simulink model "flightControlSystem"  (R2022b)
settings: Solver=ode3  StartTime=0  StopTime=TFinal  FixedStep=Ts  RelTol=1e-3  EnableMultiTasking=on
model workspace (MAT data in the model file):
  D_gain = 0.03
  I_gain = 1.9
  PD_gain = 4e-05
  P_gain = 6
  case0_gain = 0.999
  en = 0.4
  kado_delay = 20
  last_gain = 0.0008
  ririku = 400
  start = 1400
undefined symbols (not defined in the file): codertarget, Controller, DiscIntNeverNeededParam, Discrete, Estimator, g, gray, init, Sensors, Time, Ts, var_acc_angle_N, var_bias_gyr_N, var_gyro_p_N, Vehicle
libraries: simulink x80, visionstatistics x8, sldvlib x7, slpidlib x4, ctrlSharedLib x4, sharedtransform x3, dspstat3 x2, parrotlib x1
(part 2 of 3)

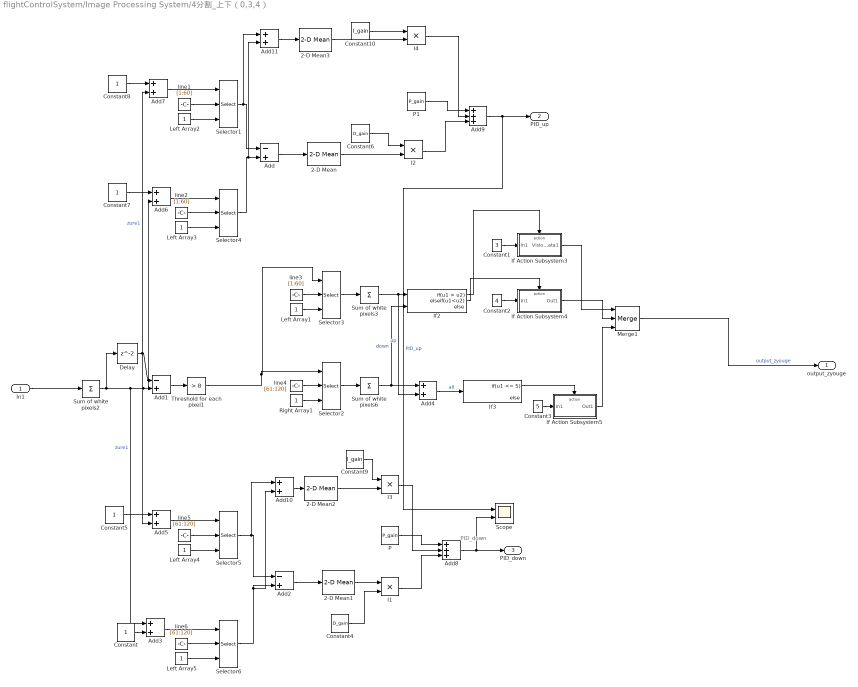
== system flightControlSystem/Image Processing System/4分割_上下（0,3,4） ==
  note: PID_down
  In1 : Inport
  2-D Mean{,1..3} (4 alike) : visionstatistics/2-D Mean  run=off  reset_popup=None  directionMode=Entire input  dimension=1  treatSBRowAsCol=on  outputLastDataTypeStr=Inherit: Same as accumulator  accumMode=Binary point scaling  accumWordLength=32  accumFracLength=0  accumLastDataTypeStr=fixdt([],32,0)  roiEnable=off  roiType=Rectangles  roiPortion=Entire ROI  roiOutput=Individual statistics for each ROI  roiFlag=off  roundingMode=Floor  overflowMode=off  accumDataTypeStr=fixdt([],32,0)  outputDataTypeStr=Inherit: Same as accumulator  outputMin=[]  outputMax=[]
  Add : Sum  Inputs=-+
  Add1 : Sum  Inputs=-+  SaturateOnIntegerOverflow=on
  Add{3..7,10..11} (7 alike) : Sum
  Add2 : Sum  Inputs=-+
  Add8 : Sum  Inputs=+++
  Add9 : Sum  Inputs=+++
  Constant{,5,7..8} (4 alike) : Constant
  Constant1 : Constant  Value=3
  Constant10 : Constant  Value=I_gain
  Constant2 : Constant  Value=4
  Constant3 : Constant  Value=5
  Constant4 : Constant  Value=D_gain
  Constant6 : Constant  Value=D_gain
  Constant9 : Constant  Value=I_gain
  Delay : Delay
  I{1..4} (4 alike) : Product
  If Action Subsystem3 : Subsystem  TreatAsAtomicUnit=on
  If Action Subsystem4 : Subsystem  TreatAsAtomicUnit=on
  If Action Subsystem5 : Subsystem  TreatAsAtomicUnit=on
  If2 : If  NumInputs=2  IfExpression=u1 > u2  ElseIfExpressions=u1<u2
  If3 : If  IfExpression=u1 <= 5
  Left Array{1..5} (5 alike) : Constant  OutMin=[1]
  Merge1 : Merge  Inputs=3  InitialOutput=[0]
  P : Constant  Value=P_gain
  P1 : Constant  Value=P_gain
  Right Array1 : Constant  OutMin=[1]
  Scope : Scope  NumInputPorts=2
  Selector{1..6} (6 alike) : Selector  NumberOfDimensions=2  InputPortWidth=3  IndexOptions=Index vector (port),Index vector (port)  Indices=[1 3],1  OutputSizes=1,1
  Sum of white pixels2 : Sum  Inputs=+  CollapseMode=Specified dimension  CollapseDim=2  OutDataTypeStr=uint16
  Sum of white pixels3 : Sum  Inputs=+  OutDataTypeStr=uint16
  Sum of white pixels6 : Sum  Inputs=+  OutDataTypeStr=uint16
  Threshold for each pixel1 : simulink/Logic and Bit Operations/Compare To Constant  relop=>  const=8  OutDataTypeStr=boolean
  line1 : Constant  Value=[1:60]
  line2 : Constant  Value=[1:60]
  line3 : Constant  Value=[1:60]
  line4 : Constant  Value=[61:120]
  line5 : Constant  Value=[61:120]
  line6 : Constant  Value=[61:120]
  output_zyouge : Outport
  PID_up : Outport  Port=2
  PID_down : Outport  Port=3
  wires:
  Constant3/1 -> If Action Subsystem5/1(In1)
  Merge1/1 -> output_zyouge/1  "output_zyouge"
  Add1/1 -> Threshold for each pixel1/1
  line3/1 -> Selector3/2
  Left Array1/1 -> Selector3/3
  Right Array1/1 -> Selector2/3
  If3/1 -> If Action Subsystem5/Action
  Sum of white pixels3/1 -> If2/1, Add4/1  "up"
  If Action Subsystem5/1(Out1) -> Merge1/3
  Sum of white pixels6/1 -> Add4/2, If2/2  "down"
  Threshold for each pixel1/1 -> Selector2/1, Selector3/1
  line4/1 -> Selector2/2
  If2/1 -> If Action Subsystem3/Action
  Constant2/1 -> If Action Subsystem4/1(In1)
  If2/2 -> If Action Subsystem4/Action
  Selector3/1 -> Sum of white pixels3/1
  If Action Subsystem4/1(Out1) -> Merge1/2
  If Action Subsystem3/1(Vision-based Data1) -> Merge1/1
  Add4/1 -> If3/1  "all"
  Constant1/1 -> If Action Subsystem3/1(In1)
  In1/1 -> Sum of white pixels2/1
  Constant6/1 -> I2/1
  Selector2/1 -> Sum of white pixels6/1
  Constant4/1 -> I1/2
  2-D Mean/1 -> I2/2
  2-D Mean1/1 -> I1/1
  Left Array2/1 -> Selector1/3
  line1/1 -> Selector1/2
  Left Array3/1 -> Selector4/3
  line2/1 -> Selector4/2
  Selector1/1 -> Add11/1, Add/1
  Selector4/1 -> Add11/2, Add/2
  Add/1 -> 2-D Mean/1
  Sum of white pixels2/1 -> Delay/1, Add3/1, Add6/2, Add1/2  "zure1"
  Left Array5/1 -> Selector6/3
  Selector6/1 -> Add10/2, Add2/2
  Selector5/1 -> Add10/1, Add2/1
  Left Array4/1 -> Selector5/3
  Delay/1 -> Add7/2, Add5/2, Add1/1  "zure1"
  line5/1 -> Selector5/2
  line6/1 -> Selector6/2
  Add2/1 -> 2-D Mean1/1
  Add3/1 -> Selector6/1
  Constant/1 -> Add3/2
  Add5/1 -> Selector5/1
  Constant5/1 -> Add5/1
  Add6/1 -> Selector4/1
  Constant7/1 -> Add6/1
  Add7/1 -> Selector1/1
  Constant8/1 -> Add7/1
  Add8/1 -> Scope/2, PID_down/1
  P/1 -> Add8/1
  I1/1 -> Add8/3
  Add9/1 -> Scope/1, PID_up/1  "PID_up"
  P1/1 -> Add9/1
  Add10/1 -> 2-D Mean2/1
  2-D Mean2/1 -> I3/2
  Constant9/1 -> I3/1
  I3/1 -> Add8/2
  Add11/1 -> 2-D Mean3/1
  2-D Mean3/1 -> I4/2
  Constant10/1 -> I4/1
  I4/1 -> Add9/2
  I2/1 -> Add9/3

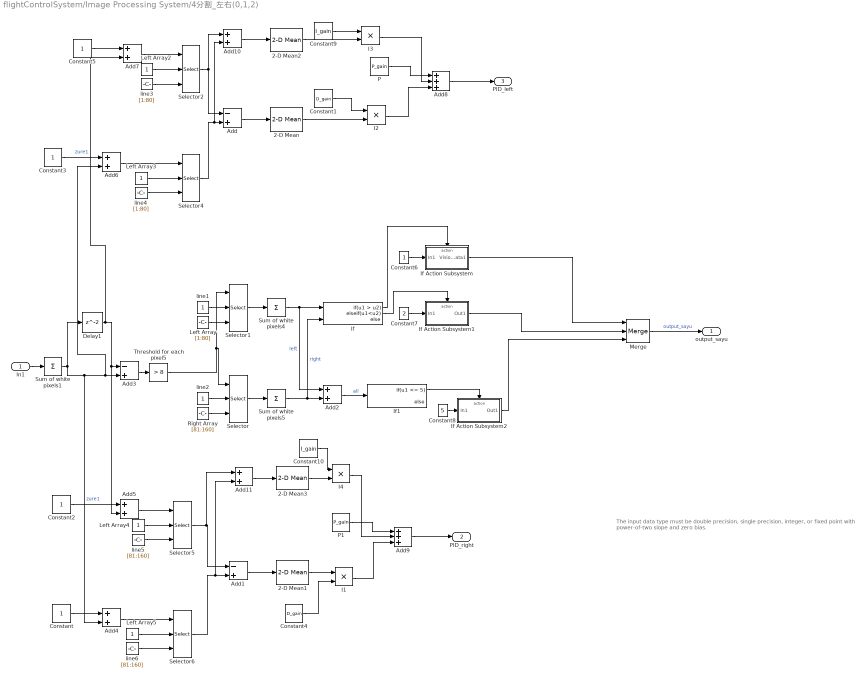
== system flightControlSystem/Image Processing System/4分割_左右(0,1,2) ==
  note: The input data type must be double precision, single precision, integer, or fixed point with power-of-two slope and zero bias.
  In1 : Inport
  2-D Mean{,1..3} (4 alike) : visionstatistics/2-D Mean  run=off  reset_popup=None  directionMode=Entire input  dimension=1  treatSBRowAsCol=on  outputLastDataTypeStr=Inherit: Same as accumulator  accumMode=Binary point scaling  accumWordLength=32  accumFracLength=0  accumLastDataTypeStr=fixdt([],32,0)  roiEnable=off  roiType=Rectangles  roiPortion=Entire ROI  roiOutput=Individual statistics for each ROI  roiFlag=off  roundingMode=Floor  overflowMode=off  accumDataTypeStr=fixdt([],32,0)  outputDataTypeStr=Inherit: Same as accumulator  outputMin=[]  outputMax=[]
  Add : Sum  Inputs=-+
  Add1 : Sum  Inputs=-+
  Add{2,4..7,10..11} (7 alike) : Sum
  Add3 : Sum  Inputs=-+  SaturateOnIntegerOverflow=on
  Add8 : Sum  Inputs=+++
  Add9 : Sum  Inputs=+++
  Constant{,2..3,5..6} (5 alike) : Constant
  Constant1 : Constant  Value=D_gain
  Constant10 : Constant  Value=I_gain
  Constant4 : Constant  Value=D_gain
  Constant7 : Constant  Value=2
  Constant8 : Constant  Value=5
  Constant9 : Constant  Value=I_gain
  Delay1 : Delay
  I{1..4} (4 alike) : Product
  If : If  NumInputs=2  IfExpression=u1 > u2  ElseIfExpressions=u1<u2
  If Action Subsystem : Subsystem  TreatAsAtomicUnit=on
  If Action Subsystem1 : Subsystem  TreatAsAtomicUnit=on
  If Action Subsystem2 : Subsystem  TreatAsAtomicUnit=on
  If1 : If  IfExpression=u1 <= 5
  Left Array : Constant  Value=[1:80]  OutMin=[1]
  Left Array{2..5} (4 alike) : Constant  OutMin=[1]
  Merge : Merge  Inputs=3  InitialOutput=[0]
  P : Constant  Value=P_gain
  P1 : Constant  Value=P_gain
  Right Array : Constant  Value=[81:160]  OutMin=[1]
  Selector{,1..2,4..6} (6 alike) : Selector  NumberOfDimensions=2  InputPortWidth=3  IndexOptions=Index vector (port),Index vector (port)  Indices=[1 3],1  OutputSizes=1,1
  Sum of white pixels1 : Sum  Inputs=+  CollapseMode=Specified dimension  OutDataTypeStr=uint16
  Sum of white pixels4 : Sum  Inputs=+  OutDataTypeStr=uint16
  Sum of white pixels5 : Sum  Inputs=+  OutDataTypeStr=uint16
  Threshold for each pixel5 : simulink/Logic and Bit Operations/Compare To Constant  relop=>  const=8  OutDataTypeStr=boolean
  line1 : Constant
  line2 : Constant
  line3 : Constant  Value=[1:80]
  line4 : Constant  Value=[1:80]
  line5 : Constant  Value=[81:160]
  line6 : Constant  Value=[81:160]
  output_sayu : Outport
  PID_right : Outport  Port=2
  PID_left : Outport  Port=3
  wires:
  If1/1 -> If Action Subsystem2/Action
  Sum of white pixels5/1 -> Add2/2, If/2  "right"
  Constant7/1 -> If Action Subsystem1/1(In1)
  Add3/1 -> Threshold for each pixel5/1
  If Action Subsystem2/1(Out1) -> Merge/3
  line1/1 -> Selector1/2
  If Action Subsystem/1(Vision-based Data1) -> Merge/1
  Right Array/1 -> Selector/3
  Sum of white pixels4/1 -> If/1, Add2/1  "left"
  Threshold for each pixel5/1 -> Selector1/1, Selector/1
  If/1 -> If Action Subsystem/Action
  If/2 -> If Action Subsystem1/Action
  If Action Subsystem1/1(Out1) -> Merge/2
  Constant8/1 -> If Action Subsystem2/1(In1)
  In1/1 -> Sum of white pixels1/1
  Left Array/1 -> Selector1/3
  Constant6/1 -> If Action Subsystem/1(In1)
  line2/1 -> Selector/2
  Add2/1 -> If1/1  "all"
  Merge/1 -> output_sayu/1  "output_sayu"
  Selector1/1 -> Sum of white pixels4/1
  Selector/1 -> Sum of white pixels5/1
  Add/1 -> 2-D Mean/1
  2-D Mean/1 -> I2/2
  Selector4/1 -> Add10/2, Add/2
  Selector2/1 -> Add10/1, Add/1
  Constant1/1 -> I2/1
  Sum of white pixels1/1 -> Add4/2, Add6/2, Add3/2, Delay1/1  "zure1"
  Add1/1 -> 2-D Mean1/1
  Selector6/1 -> Add11/2, Add1/2
  Selector5/1 -> Add11/1, Add1/1
  Delay1/1 -> Add7/2, Add5/2, Add3/1  "zure1"
  2-D Mean1/1 -> I1/1
  Constant4/1 -> I1/2
  Left Array3/1 -> Selector4/2
  line4/1 -> Selector4/3
  Left Array2/1 -> Selector2/2
  line3/1 -> Selector2/3
  Left Array4/1 -> Selector5/2
  line5/1 -> Selector5/3
  Left Array5/1 -> Selector6/2
  line6/1 -> Selector6/3
  Add4/1 -> Selector6/1
  Constant/1 -> Add4/1
  Add5/1 -> Selector5/1
  Constant2/1 -> Add5/1
  Add6/1 -> Selector4/1
  Constant3/1 -> Add6/1
  Add7/1 -> Selector2/1
  Constant5/1 -> Add7/1
  I2/1 -> Add8/3
  Add8/1 -> PID_left/1
  P/1 -> Add8/1
  I1/1 -> Add9/3
  Add9/1 -> PID_right/1
  P1/1 -> Add9/1
  Add10/1 -> 2-D Mean2/1
  2-D Mean2/1 -> I3/2
  Constant9/1 -> I3/1
  I3/1 -> Add8/2
  Add11/1 -> 2-D Mean3/1
  2-D Mean3/1 -> I4/2
  Constant10/1 -> I4/1
  I4/1 -> Add9/2

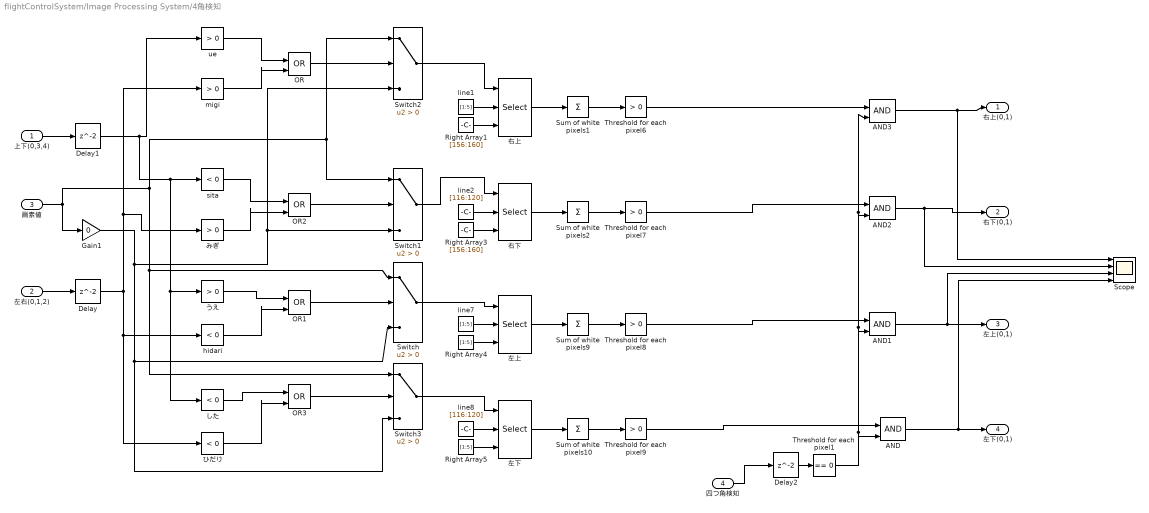
== system flightControlSystem/Image Processing System/4角検知 ==
  上下(0,3,4) : Inport
  左右(0,1,2) : Inport  Port=2
  画素値 : Inport  Port=3
  四つ角検知 : Inport  Port=4
  AND{,1..3} (4 alike) : Logic  IconShape=distinctive  AllPortsSameDT=off  OutDataTypeStr=boolean
  Delay : Delay
  Delay1 : Delay
  Delay2 : Delay
  Gain1 : Gain  Gain=0
  OR{,1..3} (4 alike) : Logic  Operator=OR  IconShape=distinctive  AllPortsSameDT=off  OutDataTypeStr=boolean
  Right Array1 : Constant  Value=[156:160]  OutMin=[1]
  Right Array3 : Constant  Value=[156:160]  OutMin=[1]
  Right Array4 : Constant  Value=[1:5]  OutMin=[1]
  Right Array5 : Constant  Value=[1:5]  OutMin=[1]
  Scope : Scope  NumInputPorts=4
  Sum of white pixels{1..2,9..10} (4 alike) : Sum  Inputs=+  OutDataTypeStr=uint16
  Switch{,1..3} (4 alike) : Switch  Criteria=u2 > Threshold  SaturateOnIntegerOverflow=off  InputSameDT=off
  Threshold for each pixel1 : simulink/Logic and Bit Operations/Compare To Constant  relop===  const=0  OutDataTypeStr=boolean
  Threshold for each pixel{6..9} (4 alike) : simulink/Logic and Bit Operations/Compare To Constant  relop=>  const=0  OutDataTypeStr=boolean
  hidari : simulink/Logic and Bit Operations/Compare To Constant  relop=<  const=0  OutDataTypeStr=boolean
  line1 : Constant  Value=[1:5]
  line2 : Constant  Value=[116:120]
  line7 : Constant  Value=[1:5]
  line8 : Constant  Value=[116:120]
  migi : simulink/Logic and Bit Operations/Compare To Constant  relop=>  const=0  OutDataTypeStr=boolean
  sita : simulink/Logic and Bit Operations/Compare To Constant  relop=<  const=0  OutDataTypeStr=boolean
  ue : simulink/Logic and Bit Operations/Compare To Constant  relop=>  const=0  OutDataTypeStr=boolean
  うえ : simulink/Logic and Bit Operations/Compare To Constant  relop=>  const=0  OutDataTypeStr=boolean
  した : simulink/Logic and Bit Operations/Compare To Constant  relop=<  const=0  OutDataTypeStr=boolean
  ひだり : simulink/Logic and Bit Operations/Compare To Constant  relop=<  const=0  OutDataTypeStr=boolean
  みぎ : simulink/Logic and Bit Operations/Compare To Constant  relop=>  const=0  OutDataTypeStr=boolean
  右上 : Selector  NumberOfDimensions=2  InputPortWidth=3  IndexOptions=Index vector (port),Index vector (port)  Indices=[1 3],1  OutputSizes=1,1
  右下 : Selector  NumberOfDimensions=2  InputPortWidth=3  IndexOptions=Index vector (port),Index vector (port)  Indices=[1 3],1  OutputSizes=1,1
  左上 : Selector  NumberOfDimensions=2  InputPortWidth=3  IndexOptions=Index vector (port),Index vector (port)  Indices=[1 3],1  OutputSizes=1,1
  左下 : Selector  NumberOfDimensions=2  InputPortWidth=3  IndexOptions=Index vector (port),Index vector (port)  Indices=[1 3],1  OutputSizes=1,1
  右上(0,1) : Outport
  右下(0,1) : Outport  Port=2
  左上(0,1) : Outport  Port=3
  左下(0,1) : Outport  Port=4
  wires:
  左下/1 -> Sum of white pixels10/1
  line2/1 -> 右下/2
  Right Array5/1 -> 左下/3
  line8/1 -> 左下/2
  Right Array3/1 -> 右下/3
  line1/1 -> 右上/2
  右上/1 -> Sum of white pixels1/1
  Right Array4/1 -> 左上/3
  右下/1 -> Sum of white pixels2/1
  Sum of white pixels9/1 -> Threshold for each pixel8/1
  左上/1 -> Sum of white pixels9/1
  Sum of white pixels1/1 -> Threshold for each pixel6/1
  Right Array1/1 -> 右上/3
  line7/1 -> 左上/2
  Sum of white pixels2/1 -> Threshold for each pixel7/1
  Threshold for each pixel9/1 -> AND/1
  Sum of white pixels10/1 -> Threshold for each pixel9/1
  Threshold for each pixel7/1 -> AND2/1
  Threshold for each pixel8/1 -> AND1/1
  Threshold for each pixel6/1 -> AND3/1
  AND3/1 -> Scope/1, 右上(0,1)/1
  AND2/1 -> Scope/2, 右下(0,1)/1
  AND1/1 -> Scope/3, 左上(0,1)/1
  AND/1 -> Scope/4, 左下(0,1)/1
  画素値/1 -> Switch3/1, Switch/1, Switch1/1, Switch2/1, Gain1/1
  左右(0,1,2)/1 -> Delay/1
  Switch/1 -> 左上/1
  Switch1/1 -> 右下/1
  ue/1 -> OR/1
  migi/1 -> OR/2
  OR/1 -> Switch2/2
  Switch2/1 -> 右上/1
  上下(0,3,4)/1 -> Delay1/1
  Switch3/1 -> 左下/1
  Delay1/1 -> ue/1, した/1, うえ/1, sita/1
  Delay/1 -> みぎ/1, migi/1, hidari/1, ひだり/1
  Gain1/1 -> Switch1/3, Switch2/3, Switch/3, Switch3/3
  OR2/1 -> Switch1/2
  OR1/1 -> Switch/2
  OR3/1 -> Switch3/2
  ひだり/1 -> OR3/2
  した/1 -> OR3/1
  hidari/1 -> OR1/2
  うえ/1 -> OR1/1
  みぎ/1 -> OR2/2
  sita/1 -> OR2/1
  四つ角検知/1 -> Delay2/1
  Delay2/1 -> Threshold for each pixel1/1
  Threshold for each pixel1/1 -> AND1/2, AND3/2, AND2/2, AND/2

== system flightControlSystem/Image Processing System/If Action Subsystem ==
  In1 : Inport
  Action Port : ActionPort  ActionPortLabel=if(u1 == 0 & u2==5)
  Out1 : Outport
  wires:
  In1/1 -> Out1/1

== system flightControlSystem/Image Processing System/If Action Subsystem1 ==
  In1 : Inport
  Action Port : ActionPort  ActionPortLabel=else
  Out1 : Outport
  wires:
  In1/1 -> Out1/1

== system flightControlSystem/Image Processing System/If Action Subsystem2 ==
  In1 : Inport  OutDataTypeStr=double
  Action Port : ActionPort  ActionPortLabel=if(u1 == 0 & u2==5)
  Out1 : Outport
  wires:
  In1/1 -> Out1/1

== system flightControlSystem/Image Processing System/If Action Subsystem3 ==
  In1 : Inport
  Action Port : ActionPort  ActionPortLabel=else
  Out1 : Outport
  wires:
  In1/1 -> Out1/1

== system flightControlSystem/Image Processing System/Switch Case Action Subsystem ==
  In1 : Inport
  Action Port : ActionPort  ActionPortLabel=case [ 0 ]:
  Out1 : Outport
  wires:
  In1/1 -> Out1/1

== system flightControlSystem/Image Processing System/Switch Case Action Subsystem1 ==
  In1 : Inport
  Action Port : ActionPort  ActionPortLabel=case [ 7 ]:
  Out1 : Outport
  wires:
  In1/1 -> Out1/1

== system flightControlSystem/Image Processing System/Switch Case Action Subsystem2 ==
  In1 : Inport
  Action Port : ActionPort  ActionPortLabel=case [ 3 ]:
  Out1 : Outport
  wires:
  In1/1 -> Out1/1

== system flightControlSystem/Image Processing System/Switch Case Action Subsystem3 ==
  In1 : Inport
  Action Port : ActionPort  ActionPortLabel=case [ 4 ]:
  Out1 : Outport
  wires:
  In1/1 -> Out1/1

== system flightControlSystem/Image Processing System/Switch Case Action Subsystem4 ==
  In1 : Inport
  Action Port : ActionPort  ActionPortLabel=case [ 3 ]:
  Out1 : Outport
  wires:
  In1/1 -> Out1/1

== system flightControlSystem/Image Processing System/Switch Case Action Subsystem5 ==
  In1 : Inport
  Action Port : ActionPort  ActionPortLabel=case [ 2 ]:
  Out1 : Outport
  wires:
  In1/1 -> Out1/1

== system flightControlSystem/Image Processing System/Switch Case Action Subsystem6 ==
  In1 : Inport
  Action Port : ActionPort  ActionPortLabel=case [ 1 ]:
  Out1 : Outport
  wires:
  In1/1 -> Out1/1

== system flightControlSystem/Image Processing System/Switch Case Action Subsystem7 ==
  In1 : Inport
  Action Port : ActionPort  ActionPortLabel=case [ 0 ]:
  Out1 : Outport
  wires:
  In1/1 -> Out1/1

== system flightControlSystem/Image Processing System/外枠検知 ==
  In1 : Inport
  Right Array1 : Constant  Value=[1:160]  OutMin=[1]
  Right Array3 : Constant  Value=[1:160]  OutMin=[1]
  Right Array4 : Constant  Value=[120:160]  OutMin=[1]
  Right Array5 : Constant  Value=[1:40]  OutMin=[1]
  Sum of white pixels{1..2,9..10} (4 alike) : Sum  Inputs=+  OutDataTypeStr=uint16
  Threshold for each pixel{6..9} (4 alike) : simulink/Logic and Bit Operations/Compare To Constant  relop=<=  const=5  OutDataTypeStr=boolean
  line1 : Constant  Value=[1:30]
  line2 : Constant  Value=[90:120]
  line7 : Constant  Value=[1:120]
  line8 : Constant  Value=[1:120]
  上上 : Selector  NumberOfDimensions=2  InputPortWidth=3  IndexOptions=Index vector (port),Index vector (port)  Indices=[1 3],1  OutputSizes=1,1
  下下 : Selector  NumberOfDimensions=2  InputPortWidth=3  IndexOptions=Index vector (port),Index vector (port)  Indices=[1 3],1  OutputSizes=1,1
  右右 : Selector  NumberOfDimensions=2  InputPortWidth=3  IndexOptions=Index vector (port),Index vector (port)  Indices=[1 3],1  OutputSizes=1,1
  左左 : Selector  NumberOfDimensions=2  InputPortWidth=3  IndexOptions=Index vector (port),Index vector (port)  Indices=[1 3],1  OutputSizes=1,1
  y : Outport
  y1 : Outport  Port=2
  y2 : Outport  Port=3
  y3 : Outport  Port=4
  wires:
  line1/1 -> 上上/2
  上上/1 -> Sum of white pixels1/1
  Sum of white pixels1/1 -> Threshold for each pixel6/1
  In1/1 -> 右右/1, 左左/1, 下下/1, 上上/1
  Sum of white pixels2/1 -> Threshold for each pixel7/1
  Sum of white pixels9/1 -> Threshold for each pixel8/1
  左左/1 -> Sum of white pixels10/1
  Threshold for each pixel6/1 -> y/1
  line8/1 -> 左左/2
  line7/1 -> 右右/2
  Sum of white pixels10/1 -> Threshold for each pixel9/1
  右右/1 -> Sum of white pixels9/1
  Right Array1/1 -> 上上/3
  Right Array4/1 -> 右右/3
  line2/1 -> 下下/2
  Threshold for each pixel7/1 -> y1/1
  下下/1 -> Sum of white pixels2/1
  Threshold for each pixel9/1 -> y2/1
  Right Array3/1 -> 下下/3
  Right Array5/1 -> 左左/3
  Threshold for each pixel8/1 -> y3/1

== system flightControlSystem/Image Processing System/論理回路 ==
  In1 : Inport
  In2 : Inport  Port=2
  In3 : Inport  Port=3
  In4 : Inport  Port=4
  AND{,1..3} (4 alike) : Logic  Inputs=4  IconShape=distinctive  AllPortsSameDT=off  OutDataTypeStr=boolean
  NOT{,1..3} (4 alike) : Logic  Operator=NOT  IconShape=distinctive  AllPortsSameDT=off  OutDataTypeStr=boolean
  OR : Logic  Operator=OR  Inputs=4  IconShape=distinctive  AllPortsSameDT=off  OutDataTypeStr=boolean
  Out1 : Outport
  wires:
  In1/1 -> AND/1, NOT/1
  In2/1 -> AND1/2, NOT1/1
  In3/1 -> AND2/3, NOT2/1
  In4/1 -> AND3/4, NOT3/1
  NOT/1 -> AND2/1, AND1/1, AND3/1
  NOT1/1 -> AND3/2, AND2/2, AND/2
  NOT2/1 -> AND3/3, AND/3, AND1/3
  NOT3/1 -> AND2/4, AND1/4, AND/4
  AND/1 -> OR/1
  AND1/1 -> OR/2
  AND2/1 -> OR/3
  AND3/1 -> OR/4
  OR/1 -> Out1/1

== system flightControlSystem/Control System/Controller/Altitude Controller ==
  note: PID Controller for Altitude
  note: ALTITUDE CONTROLLER
  states_estim : Inport
  PosZ : Inport  Port=2
  takeoff_flag : Inport  Port=3
  Bus Selector1 : BusSelector  OutputSignals=Z,dz
  Compare To Constant : simulink/Logic and Bit Operations/Compare To Constant  relop=<  const=100  OutDataTypeStr=boolean
  Counter Free-Running : simulink/Sources/Counter Free-Running  NumBits=16  tsamp=-1
  D_z1 : Gain  Gain=0.5  ParamDataTypeStr=single  OutDataTypeStr=single  SaturateOnIntegerOverflow=on
  Discrete-Time Integrator : DiscreteIntegrator  ExternalReset=falling  SampleTime=Ts  LimitOutput=on  UpperSaturationLimit=2  LowerSaturationLimit=-2  ICPrevOutput=DiscIntNeverNeededParam  ICPrevScaledInput=DiscIntNeverNeededParam
  I_pr : Gain  Gain=0.24
  P_z1 : Gain  Gain=0.8  ParamDataTypeStr=single  OutDataTypeStr=single  SaturateOnIntegerOverflow=on
  SaturationThrust1 : Saturate  UpperLimit=4*Controller.totalThrustMaxRelative*Controller.motorsThrustPerMotorMax  LowerLimit=-4*Controller.totalThrustMaxRelative*Controller.motorsThrustPerMotorMax  OutDataTypeStr=single
  Sum1 : Sum  Inputs=++-  AccumDataTypeStr=single  OutDataTypeStr=single  SaturateOnIntegerOverflow=on
  Sum2 : Sum  Inputs=+-|  AccumDataTypeStr=single  OutDataTypeStr=single  SaturateOnIntegerOverflow=on
  Sum5 : Sum  Inputs=++|  AccumDataTypeStr=single  OutDataTypeStr=single  SaturateOnIntegerOverflow=on
  TakeoffOrControl_Switch1 : Switch  Criteria=u2 > Threshold  SaturateOnIntegerOverflow=off  InputSameDT=off
  Terminator : Terminator
  takeoff_gain1 : Gain  Gain=Controller.takeoffGain  ParamDataTypeStr=single  OutDataTypeStr=single  SaturateOnIntegerOverflow=on
  w1 : Constant  Value=-g*Vehicle.Airframe.mass  OutDataTypeStr=single  SampleTime=Ts
  altitude_cmd : Outport  VectorParamsAs1DForOutWhenUnconnected=off
  wires:
  TakeoffOrControl_Switch1/1 -> Sum5/2
  Discrete-Time Integrator/1 -> Sum1/1
  PosZ/1 -> Sum2/1
  takeoff_flag/1 -> Terminator/1
  w1/1 -> Sum5/1, takeoff_gain1/1  "Feed forward term to  compensate for gravity"
  P_z1/1 -> Sum1/2
  Counter Free-Running/1 -> Compare To Constant/1
  Bus Selector1/2 -> D_z1/1  "<dz>"
  Sum5/1 -> SaturationThrust1/1
  Bus Selector1/1 -> Sum2/2  "<Z>"
  D_z1/1 -> Sum1/3  "dz"
  Sum1/1 -> TakeoffOrControl_Switch1/3
  Compare To Constant/1 -> Discrete-Time Integrator/2, TakeoffOrControl_Switch1/2
  takeoff_gain1/1 -> TakeoffOrControl_Switch1/1
  states_estim/1 -> Bus Selector1/1
  Sum2/1 -> I_pr/1, P_z1/1  "pitch/roll error"
  I_pr/1 -> Discrete-Time Integrator/1
  SaturationThrust1/1 -> altitude_cmd/1

== system flightControlSystem/Control System/Controller/Attitude Controller ==
  note: Inner loop PID
      | controls angular velocity
  note: Outer Proportional loop
      | controls the pitch and roll angle
  note: ATTITUDE CONTROL
  refAttitude : Inport
  states_estim : Inport  Port=2
  Angle control loop : slpidlib/PID Controller  Controller=P  Form=Parallel  TimeDomain=Discrete-time  UseExternalTs=off  SampleTime=Ts  IntegratorMethod=Forward Euler  FilterMethod=Forward Euler  ControllerParametersSource=internal  P=4  I=1  UseKiTs=off  D=0  N=100  UseFilter=on  TunerSelectOption=Transfer Function Based (PID Tuner App)  InitialConditionSource=internal  InitialConditionForIntegrator=0  InitialConditionForFilter=0  DifferentiatorICPrevScaledInput=0  ExternalReset=none  TrackingMode=off  Kt=1  LimitOutput=off  SatLimitsSource=internal  UpperSaturationLimit=inf  LowerSaturationLimit=-inf  LinearizeAsGain=on  AntiWindupMode=none  Kb=1  LimitIntegrator=off  UpperIntegratorSaturationLimit=inf  LowerIntegratorSaturationLimit=-inf  POutMin=[]  POutMax=[]  IOutMin=[]  IOutMax=[]  DOutMin=[]  DOutMax=[]  NOutMin=[]  NOutMax=[]  SumOutMin=[]  SumOutMax=[]  SaturationOutMin=[]  SaturationOutMax=[]  PParamMin=[]  PParamMax=[]  IParamMin=[]  IParamMax=[]  DParamMin=[]  DParamMax=[]  NParamMin=[]  NParamMax=[]  KbParamMin=[]  KbParamMax=[]  KtParamMin=[]  KtParamMax=[]  KbOutMin=[]  KbOutMax=[]  KtOutMin=[]  KtOutMax=[]  IntegratorOutMin=[]  IntegratorOutMax=[]  FilterOutMin=[]  FilterOutMax=[]  SumI1OutMin=[]  SumI1OutMax=[]  SumI2OutMin=[]  SumI2OutMax=[]  SumI3OutMin=[]  SumI3OutMax=[]  SumI4OutMin=[]  SumI4OutMax=[]  SumDOutMin=[]  SumDOutMax=[]  DifferentiatorOutMin=[]  DifferentiatorOutMax=[]  FilterDiffOutCoefMin=[]  FilterDiffOutCoefMax=[]  ReciprocalOutMin=[]  ReciprocalOutMax=[]  SumDenOutMin=[]  SumDenOutMax=[]  SumNumOutMin=[]  SumNumOutMax=[]  DivideOutMin=[]  DivideOutMax=[]  UdiffTsProdOutMin=[]  UdiffTsProdOutMax=[]  NTsProdOutMin=[]  NTsProdOutMax=[]  UintegralTsProdOutMin=[]  UintegralTsProdOutMax=[]  UngainTsProdOutMin=[]  UngainTsProdOutMax=[]  ClampingZeroOutDataTypeStr=Inherit: Inherit via back propagation  ClampingZeroOutMin=[]  ClampingZeroOutMax=[]  FilterDenConstantOutDataTypeStr=Inherit: Inherit via back propagation  FilterDenConstantOutMin=[]  FilterDenConstantOutMax=[]  PCopyOutDataTypeStr=Inherit: Inherit via back propagation  PCopyOutMin=[]  PCopyOutMax=[]  NCopyOutDataTypeStr=Inherit: Inherit via back propagation  NCopyOutMin=[]  NCopyOutMax=[]  IntegratorContinuousStateAttributes=''  IntegratorStateMustResolveToSignalObject=off  IntegratorRTWStateStorageClass=Auto  FilterContinuousStateAttributes=''  FilterStateMustResolveToSignalObject=off  FilterRTWStateStorageClass=Auto  ParallelPVariant=InternalParameters  IdealPVariant=Disabled  IVariant=Disabled  DVariant=Disabled  IntegratorVariant=Disabled  SatVariant=Disabled  AWVariant=Disabled  PCopyVariant=Disabled  TRVariant=Disabled  FdbkBlocksVariant=Forward  IdealPFdbkVariant=Disabled  SatFdbkVariant=Disabled  DerivativeFilterVariant=Disabled  NVariant=Disabled  NCopyVariant=Disabled_SignalSpec  FilterICVariant=Disabled  IntegratorICVariant=Disabled  ExternalResetVariant=Disabled  TRSumVariant=Passthrough  SumFdbkVariant=Disabled  SumVariant=Passthrough_P  TsampFilterVariant=InternalTs  TsampNgainVariant=Passthrough  TsampIntegralVariant=Disabled_SignalSpec  ExternalSaturationOutDataTypeStr=Inherit: Same as second input
  Angular velocity control loop : slpidlib/PID Controller  Controller=PID  Form=Parallel  TimeDomain=Discrete-time  UseExternalTs=off  SampleTime=Ts  IntegratorMethod=Forward Euler  FilterMethod=Forward Euler  ControllerParametersSource=internal  P=0.003*[1 0.81]  I=2*0.003*[1 0.81]  UseKiTs=off  D=0.003/25*[1 0.81]  N=70*[1 1]  UseFilter=on  TunerSelectOption=Transfer Function Based (PID Tuner App)  InitialConditionSource=internal  InitialConditionForIntegrator=0  InitialConditionForFilter=0  DifferentiatorICPrevScaledInput=0  ExternalReset=none  TrackingMode=off  Kt=1  LimitOutput=on  SatLimitsSource=internal  UpperSaturationLimit=0.02  LowerSaturationLimit=-0.02  LinearizeAsGain=on  AntiWindupMode=clamping  Kb=1  LimitIntegrator=off  UpperIntegratorSaturationLimit=inf  LowerIntegratorSaturationLimit=-inf  POutMin=[]  POutMax=[]  IOutMin=[]  IOutMax=[]  DOutMin=[]  DOutMax=[]  NOutMin=[]  NOutMax=[]  SumOutMin=[]  SumOutMax=[]  SaturationOutMin=[]  SaturationOutMax=[]  PParamMin=[]  PParamMax=[]  IParamMin=[]  IParamMax=[]  DParamMin=[]  DParamMax=[]  NParamMin=[]  NParamMax=[]  KbParamMin=[]  KbParamMax=[]  KtParamMin=[]  KtParamMax=[]  KbOutMin=[]  KbOutMax=[]  KtOutMin=[]  KtOutMax=[]  IntegratorOutMin=[]  IntegratorOutMax=[]  FilterOutMin=[]  FilterOutMax=[]  SumI1OutMin=[]  SumI1OutMax=[]  SumI2OutMin=[]  SumI2OutMax=[]  SumI3OutMin=[]  SumI3OutMax=[]  SumI4OutMin=[]  SumI4OutMax=[]  SumDOutMin=[]  SumDOutMax=[]  DifferentiatorOutMin=[]  DifferentiatorOutMax=[]  FilterDiffOutCoefMin=[]  FilterDiffOutCoefMax=[]  ReciprocalOutMin=[]  ReciprocalOutMax=[]  SumDenOutMin=[]  SumDenOutMax=[]  SumNumOutMin=[]  SumNumOutMax=[]  DivideOutMin=[]  DivideOutMax=[]  UdiffTsProdOutMin=[]  UdiffTsProdOutMax=[]  NTsProdOutMin=[]  NTsProdOutMax=[]  UintegralTsProdOutMin=[]  UintegralTsProdOutMax=[]  UngainTsProdOutMin=[]  UngainTsProdOutMax=[]  ClampingZeroOutDataTypeStr=Inherit: Inherit via back propagation  ClampingZeroOutMin=[]  ClampingZeroOutMax=[]  FilterDenConstantOutDataTypeStr=Inherit: Inherit via back propagation  FilterDenConstantOutMin=[]  FilterDenConstantOutMax=[]  PCopyOutDataTypeStr=Inherit: Inherit via back propagation  PCopyOutMin=[]  PCopyOutMax=[]  NCopyOutDataTypeStr=Inherit: Inherit via back propagation  NCopyOutMin=[]  NCopyOutMax=[]  IntegratorContinuousStateAttributes=''  IntegratorStateMustResolveToSignalObject=off  IntegratorRTWStateStorageClass=Auto  FilterContinuousStateAttributes=''  FilterStateMustResolveToSignalObject=off  FilterRTWStateStorageClass=Auto  ParallelPVariant=InternalParameters  IdealPVariant=Disabled  IVariant=InternalParameters  DVariant=InternalParameters  IntegratorVariant=Discrete  SatVariant=Enabled  AWVariant=DiscClampingParallel  PCopyVariant=Disabled  TRVariant=Disabled  FdbkBlocksVariant=Forward  IdealPFdbkVariant=Disabled  SatFdbkVariant=Disabled  DerivativeFilterVariant=ForwardEulerFilter  NVariant=InternalParameters  NCopyVariant=Disabled  FilterICVariant=InternalICsFilter  IntegratorICVariant=InternalICs  ExternalResetVariant=Disabled  TRSumVariant=Passthrough  SumFdbkVariant=Disabled  SumVariant=Sum_PID  TsampFilterVariant=InternalTs  TsampNgainVariant=Passthrough  TsampIntegralVariant=Passthrough  ExternalSaturationOutDataTypeStr=Inherit: Same as second input
  Bus Selector1 : BusSelector  OutputSignals=q,p
  Bus Selector3 : BusSelector  OutputSignals=pitch,roll
  Demux1 : Demux  Outputs=2
  Mux : Mux  Inputs=2
  Mux2 : Mux  Inputs=2
  Sum1 : Sum  Inputs=|+-
  Sum19 : Sum  Inputs=|+-
  tau_pitch : Outport  VectorParamsAs1DForOutWhenUnconnected=off
  tau_roll : Outport  Port=2  VectorParamsAs1DForOutWhenUnconnected=off
  wires:
  Sum1/1 -> Angular velocity control loop/1  "pitch/roll error"
  Angle control loop/1 -> Sum1/1
  Mux2/1 -> Sum1/2
  Sum19/1 -> Angle control loop/1  "pitch/roll error"
  Angular velocity control loop/1 -> Demux1/1
  Demux1/2 -> tau_roll/1  "tau_roll"
  Demux1/1 -> tau_pitch/1  "tau_pitch"
  Bus Selector3/2 -> Mux/2  "<roll>"
  Mux/1 -> Sum19/2
  refAttitude/1 -> Sum19/1
  states_estim/1 -> Bus Selector1/1, Bus Selector3/1
  Bus Selector3/1 -> Mux/1  "<pitch>"
  Bus Selector1/1 -> Mux2/1  "<q>"
  Bus Selector1/2 -> Mux2/2  "<p>"

== system flightControlSystem/Control System/Controller/ControlMixer ==
  tau_pitch : Inport
  tau_roll : Inport  Port=2
  tau_yaw : Inport  Port=3
  totalThrust : Inport  Port=4
  Add : Sum
  Manual Switch : ManualSwitch
  Mux2 : Mux
  Pitch correction : Constant  Value=0.002  OutDataTypeStr=single
  Product : Product  Multiplication=Matrix(*)  RndMeth=Zero
  TorqueTotalThrustToThrustPerMotor : Constant  Value=Controller.Q2Ts  OutDataTypeStr=single
  Variant Source : VariantSource  VariantControlMode=sim codegen switching  VariantActivationTime=update diagram analyze all choices  ShowConditionOnBlock=on
  zero correction : Constant  Value=0  OutDataTypeStr=single
  thrusts_refout : Outport  VectorParamsAs1DForOutWhenUnconnected=off
  wires:
  Product/1 -> thrusts_refout/1
  tau_roll/1 -> Mux2/4
  Add/1 -> Variant Source/2
  tau_yaw/1 -> Mux2/2
  totalThrust/1 -> Mux2/1
  TorqueTotalThrustToThrustPerMotor/1 -> Product/1
  Mux2/1 -> Product/2
  Variant Source/1 -> Mux2/3
  tau_pitch/1 -> Add/1, Variant Source/1
  Pitch correction/1 -> Manual Switch/1
  zero correction/1 -> Manual Switch/2
  Manual Switch/1 -> Add/2

== system flightControlSystem/Control System/Controller/Position Controller ==
  note: Position controller requires good estimate of Yaw orientation to work properly.
      | Incase position control is not needed, the outer loop can be removed and velocity setpoint can be given directly
  note: Inner loop controls linear velocity error
  note: Outer loop controls the position error
  posXY : Inport
  states_estim : Inport  Port=2
  Bus Selector1 : BusSelector  OutputSignals=X,Y
  Bus Selector2 : BusSelector  OutputSignals=dx,dy
  Bus Selector3 : BusSelector  OutputSignals=yaw
  Gain : Gain  Gain=[-1, 1]
  LPF 8Hz Cutoff Filter to avoid oscillations induced by position controller : DiscreteTransferFcn  Numerator=[1, 1]  Denominator=[1+1/pi/Ts/8, 1-1/pi/Ts/8]
  Mux : Mux  Inputs=2
  Mux1 : Mux  Inputs=2
  Position controller : slpidlib/PID Controller  Controller=P  Form=Parallel  TimeDomain=Discrete-time  UseExternalTs=off  SampleTime=Ts  IntegratorMethod=Forward Euler  FilterMethod=Forward Euler  ControllerParametersSource=internal  P=0.7  I=0.1  UseKiTs=off  D=0  N=100  UseFilter=on  TunerSelectOption=Transfer Function Based (PID Tuner App)  InitialConditionSource=internal  InitialConditionForIntegrator=0  InitialConditionForFilter=0  DifferentiatorICPrevScaledInput=0  ExternalReset=none  TrackingMode=off  Kt=1  LimitOutput=on  SatLimitsSource=internal  UpperSaturationLimit=0.5  LowerSaturationLimit=-0.5  LinearizeAsGain=on  AntiWindupMode=clamping  Kb=1  LimitIntegrator=off  UpperIntegratorSaturationLimit=inf  LowerIntegratorSaturationLimit=-inf  POutMin=[]  POutMax=[]  IOutMin=[]  IOutMax=[]  DOutMin=[]  DOutMax=[]  NOutMin=[]  NOutMax=[]  SumOutMin=[]  SumOutMax=[]  SaturationOutMin=[]  SaturationOutMax=[]  PParamMin=[]  PParamMax=[]  IParamMin=[]  IParamMax=[]  DParamMin=[]  DParamMax=[]  NParamMin=[]  NParamMax=[]  KbParamMin=[]  KbParamMax=[]  KtParamMin=[]  KtParamMax=[]  KbOutMin=[]  KbOutMax=[]  KtOutMin=[]  KtOutMax=[]  IntegratorOutMin=[]  IntegratorOutMax=[]  FilterOutMin=[]  FilterOutMax=[]  SumI1OutMin=[]  SumI1OutMax=[]  SumI2OutMin=[]  SumI2OutMax=[]  SumI3OutMin=[]  SumI3OutMax=[]  SumI4OutMin=[]  SumI4OutMax=[]  SumDOutMin=[]  SumDOutMax=[]  DifferentiatorOutMin=[]  DifferentiatorOutMax=[]  FilterDiffOutCoefMin=[]  FilterDiffOutCoefMax=[]  ReciprocalOutMin=[]  ReciprocalOutMax=[]  SumDenOutMin=[]  SumDenOutMax=[]  SumNumOutMin=[]  SumNumOutMax=[]  DivideOutMin=[]  DivideOutMax=[]  UdiffTsProdOutMin=[]  UdiffTsProdOutMax=[]  NTsProdOutMin=[]  NTsProdOutMax=[]  UintegralTsProdOutMin=[]  UintegralTsProdOutMax=[]  UngainTsProdOutMin=[]  UngainTsProdOutMax=[]  ClampingZeroOutDataTypeStr=Inherit: Inherit via back propagation  ClampingZeroOutMin=[]  ClampingZeroOutMax=[]  FilterDenConstantOutDataTypeStr=Inherit: Inherit via back propagation  FilterDenConstantOutMin=[]  FilterDenConstantOutMax=[]  PCopyOutDataTypeStr=Inherit: Inherit via back propagation  PCopyOutMin=[]  PCopyOutMax=[]  NCopyOutDataTypeStr=Inherit: Inherit via back propagation  NCopyOutMin=[]  NCopyOutMax=[]  IntegratorContinuousStateAttributes=''  IntegratorStateMustResolveToSignalObject=off  IntegratorRTWStateStorageClass=Auto  FilterContinuousStateAttributes=''  FilterStateMustResolveToSignalObject=off  FilterRTWStateStorageClass=Auto  ParallelPVariant=InternalParameters  IdealPVariant=Disabled  IVariant=Disabled  DVariant=Disabled  IntegratorVariant=Disabled  SatVariant=Enabled  AWVariant=Disabled  PCopyVariant=Disabled  TRVariant=Disabled  FdbkBlocksVariant=Forward  IdealPFdbkVariant=Disabled  SatFdbkVariant=Disabled  DerivativeFilterVariant=Disabled  NVariant=Disabled  NCopyVariant=Disabled_SignalSpec  FilterICVariant=Disabled  IntegratorICVariant=Disabled  ExternalResetVariant=Disabled  TRSumVariant=Passthrough  SumFdbkVariant=Disabled  SumVariant=Passthrough_P  TsampFilterVariant=InternalTs  TsampNgainVariant=Passthrough  TsampIntegralVariant=Disabled_SignalSpec  ExternalSaturationOutDataTypeStr=Inherit: Same as second input
  Position error transformation (Earth to Body frame) : MATLAB Function  TreatAsAtomicUnit=on
  Sum1 : Sum  Inputs=|+-
  Sum19 : Sum  Inputs=|+-
  Velocity controller : slpidlib/PID Controller  Controller=PI  Form=Parallel  TimeDomain=Discrete-time  UseExternalTs=off  SampleTime=Ts  IntegratorMethod=Forward Euler  FilterMethod=Forward Euler  ControllerParametersSource=internal  P=0.2  I=0.1  UseKiTs=off  D=0  N=100  UseFilter=on  TunerSelectOption=Transfer Function Based (PID Tuner App)  InitialConditionSource=internal  InitialConditionForIntegrator=0  InitialConditionForFilter=0  DifferentiatorICPrevScaledInput=0  ExternalReset=none  TrackingMode=off  Kt=1  LimitOutput=on  SatLimitsSource=internal  UpperSaturationLimit=20*pi/180  LowerSaturationLimit=-20*pi/180  LinearizeAsGain=on  AntiWindupMode=clamping  Kb=1  LimitIntegrator=off  UpperIntegratorSaturationLimit=inf  LowerIntegratorSaturationLimit=-inf  POutMin=[]  POutMax=[]  IOutMin=[]  IOutMax=[]  DOutMin=[]  DOutMax=[]  NOutMin=[]  NOutMax=[]  SumOutMin=[]  SumOutMax=[]  SaturationOutMin=[]  SaturationOutMax=[]  PParamMin=[]  PParamMax=[]  IParamMin=[]  IParamMax=[]  DParamMin=[]  DParamMax=[]  NParamMin=[]  NParamMax=[]  KbParamMin=[]  KbParamMax=[]  KtParamMin=[]  KtParamMax=[]  KbOutMin=[]  KbOutMax=[]  KtOutMin=[]  KtOutMax=[]  IntegratorOutMin=[]  IntegratorOutMax=[]  FilterOutMin=[]  FilterOutMax=[]  SumI1OutMin=[]  SumI1OutMax=[]  SumI2OutMin=[]  SumI2OutMax=[]  SumI3OutMin=[]  SumI3OutMax=[]  SumI4OutMin=[]  SumI4OutMax=[]  SumDOutMin=[]  SumDOutMax=[]  DifferentiatorOutMin=[]  DifferentiatorOutMax=[]  FilterDiffOutCoefMin=[]  FilterDiffOutCoefMax=[]  ReciprocalOutMin=[]  ReciprocalOutMax=[]  SumDenOutMin=[]  SumDenOutMax=[]  SumNumOutMin=[]  SumNumOutMax=[]  DivideOutMin=[]  DivideOutMax=[]  UdiffTsProdOutMin=[]  UdiffTsProdOutMax=[]  NTsProdOutMin=[]  NTsProdOutMax=[]  UintegralTsProdOutMin=[]  UintegralTsProdOutMax=[]  UngainTsProdOutMin=[]  UngainTsProdOutMax=[]  ClampingZeroOutDataTypeStr=Inherit: Inherit via back propagation  ClampingZeroOutMin=[]  ClampingZeroOutMax=[]  FilterDenConstantOutDataTypeStr=Inherit: Inherit via back propagation  FilterDenConstantOutMin=[]  FilterDenConstantOutMax=[]  PCopyOutDataTypeStr=Inherit: Inherit via back propagation  PCopyOutMin=[]  PCopyOutMax=[]  NCopyOutDataTypeStr=Inherit: Inherit via back propagation  NCopyOutMin=[]  NCopyOutMax=[]  IntegratorContinuousStateAttributes=''  IntegratorStateMustResolveToSignalObject=off  IntegratorRTWStateStorageClass=Auto  FilterContinuousStateAttributes=''  FilterStateMustResolveToSignalObject=off  FilterRTWStateStorageClass=Auto  ParallelPVariant=InternalParameters  IdealPVariant=Disabled  IVariant=InternalParameters  DVariant=Disabled  IntegratorVariant=Discrete  SatVariant=Enabled  AWVariant=DiscClampingParallel  PCopyVariant=Disabled  TRVariant=Disabled  FdbkBlocksVariant=Forward  IdealPFdbkVariant=Disabled  SatFdbkVariant=Disabled  DerivativeFilterVariant=Disabled  NVariant=Disabled  NCopyVariant=Disabled_SignalSpec  FilterICVariant=Disabled  IntegratorICVariant=InternalICs  ExternalResetVariant=Disabled  TRSumVariant=Passthrough  SumFdbkVariant=Disabled  SumVariant=Sum_PI  TsampFilterVariant=InternalTs  TsampNgainVariant=Passthrough  TsampIntegralVariant=Passthrough  ExternalSaturationOutDataTypeStr=Inherit: Same as second input
  pitch_roll_cmd : Outport  VectorParamsAs1DForOutWhenUnconnected=off
  wires:
  Bus Selector2/1 -> Mux1/1  "<dx>"
  states_estim/1 -> Bus Selector2/1, Bus Selector3/1, Bus Selector1/1
  Bus Selector1/1 -> Mux/1  "<X>"
  Bus Selector1/2 -> Mux/2  "<Y>"
  Bus Selector2/2 -> Mux1/2  "<dy>"
  Mux1/1 -> Sum19/2
  Sum19/1 -> Velocity controller/1
  Velocity controller/1 -> LPF 8Hz Cutoff Filter to avoid oscillations induced by position controller/1
  Gain/1 -> pitch_roll_cmd/1  "Pitch,Roll setpoint"
  LPF 8Hz Cutoff Filter to avoid oscillations induced by position controller/1 -> Gain/1
  Position controller/1 -> Sum19/1  "Velocity  setpoint"
  Mux/1 -> Sum1/2
  Sum1/1 -> Position error transformation (Earth to Body frame)/2(xy_err_earth)
  Position error transformation (Earth to Body frame)/1(xy_err_body) -> Position controller/1
  posXY/1 -> Sum1/1  "Position setpoint"
  Bus Selector3/1 -> Position error transformation (Earth to Body frame)/1(yaw)  "<yaw>"

== system flightControlSystem/Control System/Controller/Yaw Controller ==
  note: Yaw angle is not constrained between -180 to 180 degrees
  note: Yaw estimation is done solely using the gyroscope and it may drift with time.
  yaw_ref : Inport
  states_estim : Inport  Port=2
  Bus Selector1 : BusSelector  OutputSignals=r
  Bus Selector5 : BusSelector  OutputSignals=yaw
  D_yaw : Gain  Gain=0.3*0.004
  Discrete-Time Integrator : DiscreteIntegrator  gainval=1  SampleTime=-1  ICPrevOutput=DiscIntNeverNeededParam  ICPrevScaledInput=DiscIntNeverNeededParam
  I_yaw : Gain  Gain=0.002  ParamDataTypeStr=single  OutDataTypeStr=single
  P_yaw : Gain  Gain=0.004  ParamDataTypeStr=single  OutDataTypeStr=single
  Saturation : Saturate  UpperLimit=pi/180*30  LowerLimit=-pi/180*30
  Sum1 : Sum  Inputs=|+-  AccumDataTypeStr=single  OutDataTypeStr=single  SaturateOnIntegerOverflow=on
  Sum2 : Sum  Inputs=++-
  tau_yaw : Outport  VectorParamsAs1DForOutWhenUnconnected=off
  wires:
  D_yaw/1 -> Sum2/3
  P_yaw/1 -> Sum2/1
  Bus Selector1/1 -> D_yaw/1  "<r>"
  Sum1/1 -> Saturation/1
  states_estim/1 -> Bus Selector1/1, Bus Selector5/1
  Bus Selector5/1 -> Sum1/2  "<yaw>"
  yaw_ref/1 -> Sum1/1
  Sum2/1 -> tau_yaw/1
  Discrete-Time Integrator/1 -> Sum2/2
  I_yaw/1 -> Discrete-Time Integrator/1
  Saturation/1 -> P_yaw/1, I_yaw/1

== system flightControlSystem/Control System/Controller/thrustsToMotorCommands ==
  thrusts_refin : Inport
  MotorDirections : Gain  Gain=[1 -1 1 -1]
  Saturation5 : Saturate  UpperLimit=Vehicle.Motor.maxLimit  LowerLimit=Vehicle.Motor.minLimit
  ThrustToMotorCommand : Gain  Gain=-Vehicle.Motor.thrustToMotorCommand
  motors_cmdout : Outport  VectorParamsAs1DForOutWhenUnconnected=off
  wires:
  Saturation5/1 -> MotorDirections/1
  MotorDirections/1 -> motors_cmdout/1
  ThrustToMotorCommand/1 -> Saturation5/1
  thrusts_refin/1 -> ThrustToMotorCommand/1

== system flightControlSystem/Control System/Crash Predictor Flags/Geofencing error ==
  Action Port : ActionPort  ActionPortLabel=if(u1 > 0)
  Constant : Constant  OutDataTypeStr=uint8
  Out1 : Outport  VectorParamsAs1DForOutWhenUnconnected=off
  wires:
  Constant/1 -> Out1/1

== system flightControlSystem/Control System/Crash Predictor Flags/No optical flow  ==
  Action Port : ActionPort  ActionPortLabel=elseif( u3> 0)
  Constant : Constant  Value=0  OutDataTypeStr=uint8
  Out1 : Outport  VectorParamsAs1DForOutWhenUnconnected=off
  wires:
  Constant/1 -> Out1/1

== system flightControlSystem/Control System/Crash Predictor Flags/Normal condition ==
  Action Port : ActionPort  ActionPortLabel=else
  Constant : Constant  Value=0  OutDataTypeStr=uint8
  Out1 : Outport  VectorParamsAs1DForOutWhenUnconnected=off
  wires:
  Constant/1 -> Out1/1

== system flightControlSystem/Control System/Crash Predictor Flags/Ultrasound improper ==
  Action Port : ActionPort  ActionPortLabel=elseif(u4>0)
  Constant : Constant  Value=0  OutDataTypeStr=uint8
  Out1 : Outport  VectorParamsAs1DForOutWhenUnconnected=off
  wires:
  Constant/1 -> Out1/1

== system flightControlSystem/Control System/Crash Predictor Flags/estimator//Optical flow error ==
  Action Port : ActionPort  ActionPortLabel=elseif(u2 > 0)
  Constant : Constant  Value=99  OutDataTypeStr=uint8
  Out1 : Outport  VectorParamsAs1DForOutWhenUnconnected=off
  wires:
  Constant/1 -> Out1/1

== system flightControlSystem/Control System/Path Planning/Switch Case Action Subsystem1 ==
  In1 : Inport
  Action Port : ActionPort  ActionPortLabel=case [ 4 ]:
  Out1 : Outport
  wires:
  In1/1 -> Out1/1

== system flightControlSystem/Control System/Path Planning/Switch Case Action Subsystem10 ==
  In1 : Inport
  Action Port : ActionPort  ActionPortLabel=case [ 2 ]:
  Out1 : Outport
  wires:
  In1/1 -> Out1/1

== system flightControlSystem/Control System/Path Planning/Switch Case Action Subsystem11 ==
  In1 : Inport
  Action Port : ActionPort  ActionPortLabel=case [ 0 ]:
  Out1 : Outport
  wires:
  In1/1 -> Out1/1

== system flightControlSystem/Control System/Path Planning/Switch Case Action Subsystem12 ==
  In1 : Inport
  Action Port : ActionPort  ActionPortLabel=case [ 3 ]:
  Out1 : Outport
  wires:
  In1/1 -> Out1/1

== system flightControlSystem/Control System/Path Planning/Switch Case Action Subsystem13 ==
  In1 : Inport
  Action Port : ActionPort  ActionPortLabel=case [ 10 ]:
  Out1 : Outport
  wires:
  In1/1 -> Out1/1

== system flightControlSystem/Control System/Path Planning/Switch Case Action Subsystem14 ==
  In1 : Inport
  Action Port : ActionPort  ActionPortLabel=case [ 6 ]:
  Out1 : Outport
  wires:
  In1/1 -> Out1/1

== system flightControlSystem/Control System/Path Planning/Switch Case Action Subsystem15 ==
  In1 : Inport
  Action Port : ActionPort  ActionPortLabel=case [ 8 ]:
  Out1 : Outport
  wires:
  In1/1 -> Out1/1

== system flightControlSystem/Control System/Path Planning/Switch Case Action Subsystem16 ==
  In1 : Inport
  Action Port : ActionPort  ActionPortLabel=case [ 15 ]:
  Out1 : Outport
  wires:
  In1/1 -> Out1/1

== system flightControlSystem/Control System/Path Planning/Switch Case Action Subsystem17 ==
  In1 : Inport
  Action Port : ActionPort  ActionPortLabel=case [ 3 ]:
  Out1 : Outport
  wires:
  In1/1 -> Out1/1

== system flightControlSystem/Control System/Path Planning/Switch Case Action Subsystem18 ==
  In1 : Inport
  Action Port : ActionPort  ActionPortLabel=case [ 6 ]:
  Out1 : Outport
  wires:
  In1/1 -> Out1/1

== system flightControlSystem/Control System/Path Planning/Switch Case Action Subsystem19 ==
  In1 : Inport
  Action Port : ActionPort  ActionPortLabel=case [ 0 ]:
  Out1 : Outport
  wires:
  In1/1 -> Out1/1

== system flightControlSystem/Control System/Path Planning/Switch Case Action Subsystem2 ==
  In1 : Inport
  Action Port : ActionPort  ActionPortLabel=case [ 5 ]:
  Out1 : Outport
  wires:
  In1/1 -> Out1/1

== system flightControlSystem/Control System/Path Planning/Switch Case Action Subsystem20 ==
  In1 : Inport
  Action Port : ActionPort  ActionPortLabel=case [ 0 ]:
  Out1 : Outport
  wires:
  In1/1 -> Out1/1

== system flightControlSystem/Control System/Path Planning/Switch Case Action Subsystem21 ==
  In1 : Inport
  Action Port : ActionPort  ActionPortLabel=case [ 13 ]:
  Out1 : Outport
  wires:
  In1/1 -> Out1/1

== system flightControlSystem/Control System/Path Planning/Switch Case Action Subsystem22 ==
  In1 : Inport
  Action Port : ActionPort  ActionPortLabel=case [ 14 ]:
  Out1 : Outport
  wires:
  In1/1 -> Out1/1

== system flightControlSystem/Control System/Path Planning/Switch Case Action Subsystem23 ==
  In1 : Inport
  Action Port : ActionPort  ActionPortLabel=case [ 11 ]:
  Out1 : Outport
  wires:
  In1/1 -> Out1/1

== system flightControlSystem/Control System/Path Planning/Switch Case Action Subsystem24 ==
  In1 : Inport
  Action Port : ActionPort  ActionPortLabel=case [ 12 ]:
  Out1 : Outport
  wires:
  In1/1 -> Out1/1

== system flightControlSystem/Control System/Path Planning/Switch Case Action Subsystem3 ==
  In1 : Inport
  Action Port : ActionPort  ActionPortLabel=case [ 4 ]:
  Out1 : Outport
  wires:
  In1/1 -> Out1/1

== system flightControlSystem/Control System/Path Planning/Switch Case Action Subsystem4 ==
  In1 : Inport
  Action Port : ActionPort  ActionPortLabel=case [ 3 ]:
  Out1 : Outport
  wires:
  In1/1 -> Out1/1

== system flightControlSystem/Control System/Path Planning/Switch Case Action Subsystem5 ==
  In1 : Inport
  Action Port : ActionPort  ActionPortLabel=case [ 5 ]:
  Out1 : Outport
  wires:
  In1/1 -> Out1/1

== system flightControlSystem/Control System/Path Planning/Switch Case Action Subsystem6 ==
  In1 : Inport
  Action Port : ActionPort  ActionPortLabel=case [ 2 ]:
  Out1 : Outport
  wires:
  In1/1 -> Out1/1

== system flightControlSystem/Control System/Path Planning/Switch Case Action Subsystem7 ==
  In1 : Inport
  Action Port : ActionPort  ActionPortLabel=case [ 1 ]:
  Out1 : Outport
  wires:
  In1/1 -> Out1/1

== system flightControlSystem/Control System/Path Planning/Switch Case Action Subsystem8 ==
  In1 : Inport
  Action Port : ActionPort  ActionPortLabel=case [ 0 ]:
  Out1 : Outport
  wires:
  In1/1 -> Out1/1

== system flightControlSystem/Control System/Path Planning/Switch Case Action Subsystem9 ==
  In1 : Inport
  Action Port : ActionPort  ActionPortLabel=case [ 1 ]:
  Out1 : Outport
  wires:
  In1/1 -> Out1/1

== system flightControlSystem/Control System/Path Planning/最初の動きと4分割出力_上下 ==
  In1 : Inport
  外枠上下(0,5,3,4) : Inport  Port=2
  AND : Logic  IconShape=distinctive  AllPortsSameDT=off  OutDataTypeStr=boolean
  Add4 : Sum
  Constant : Constant  Value=5
  Constant6 : Constant
  Constant7 : Constant  Value=5
  Delay6 : Delay  DelayLength=1
  Gain(0,10,6,8) : Gain  Gain=2
  Switch : Switch  Criteria=u2 > Threshold  SaturateOnIntegerOverflow=off  InputSameDT=off
  Switch1 : Switch  Criteria=u2 ~= 0  SaturateOnIntegerOverflow=off  InputSameDT=off
  Switch2 : Switch  Threshold=ririku  SaturateOnIntegerOverflow=off  InputSameDT=off
  Threshold for each pixel1 : simulink/Logic and Bit Operations/Compare To Constant  relop=<  const=start  OutDataTypeStr=boolean
  Threshold for each pixel10 : simulink/Logic and Bit Operations/Compare To Constant  relop=>  const=ririku  OutDataTypeStr=boolean
  Out1 : Outport
  wires:
  Add4/1 -> Delay6/1, Threshold for each pixel1/1, Threshold for each pixel10/1, Switch2/2  "yValue"
  Threshold for each pixel10/1 -> AND/1
  Switch2/1 -> Switch/3
  外枠上下(0,5,3,4)/1 -> Switch1/1, Switch1/2
  AND/1 -> Switch/2
  Delay6/1 -> Add4/2
  Constant6/1 -> Add4/1
  Threshold for each pixel1/1 -> AND/2
  In1/1 -> Switch2/1
  Constant7/1 -> Switch2/3
  Switch/1 -> Out1/1
  Gain(0,10,6,8)/1 -> Switch/1
  Constant/1 -> Switch1/3
  Switch1/1 -> Gain(0,10,6,8)/1
